simulink model "BMS_OL_Harness_advancedcell"  (R2015b)
settings: Solver=FixedStepDiscrete  StartTime=0.0  StopTime=660  FixedStep=BMSk_stepSize  RelTol=1e-3
undefined symbols (not defined in the file): BMSc_airTemperature, BMSc_cabinTemperature, BMSk_stepSize
settings Model: PauseTimes=22  Creator=ms2zwt  LastModifiedBy=nctzv8
settings ConfigSet: Description=OpenECU configuration set for code generation under RTW-EC.
settings SolverCC: PositivePriorityOrder=on
settings DataIOCC: SaveFormat=Array  SignalLoggingSaveFormat=ModelDataLogs
settings OptimizationCC: DefaultParameterBehavior=Inlined  InlineInvariantSignals=on  ExpressionDepthLimit=2147483647  StateBitsets=on  DataBitsets=on  ZeroExternalMemoryAtStartup=off  ZeroInternalMemoryAtStartup=off  NoFixptDivByZeroProtection=on  EfficientFloat2IntCast=on  OptimizeModelRefInitCode=on  LifeSpan=1
settings DebuggingCC: SaveWithParameterizedLinksMsg=none  UnderspecifiedInitializationDetection=Classic  MergeDetectMultiDrivingBlocksExec=none  SignalResolutionControl=TryResolveAllWithWarning  MultiTaskDSMMsg=warning  MultiTaskCondExecSysMsg=none  SingleTaskRateTransMsg=error  CheckMatrixSingularityMsg=warning  VectorMatrixConversionMsg=warning  FcnCallInpInsideContextMsg=UseLocalSettings  SignalLabelMismatchMsg=warning  StateNameClashWarn=warning
settings HardwareCC: ProdBitPerPointer=32  ProdLargestAtomicInteger=Long  ProdLargestAtomicFloat=Double  ProdEndianess=BigEndian  ProdWordSize=32  ProdHWDeviceType=Freescale->32-bit PowerPC  TargetIntDivRoundTo=Zero  TargetEndianess=BigEndian  TargetHWDeviceType=Freescale->32-bit PowerPC  ProdEqTarget=off
settings RTWCC: SystemTargetFile=openecu_ert.tlc  MakeCommand=make_rtw optimized_floating_point=1  TemplateMakefile=openecu_ert_r2015b_64.tmf  Description=OpenECU Platform Target (ERT, optimised floating-point code)  RetainRTWFile=on  IncludeHyperlinkInReport=on
settings CodeAppCC: ForceParamTrailComments=on  IgnoreCustomStorageClasses=off  SimulinkDataObjDesc=on  CustomSymbolStrType=$N$R$M  InsertBlockDesc=on  InternalIdentifier=Classic
settings STFCustomTargetCC: TargetLibSuffix=.a  GenerateSampleERTMain=on  ConcurrentExecutionCompliant=off  IncludeMdlTerminateFcn=off  GeneratePreprocessorConditionals=Use local settings  CombineOutputUpdateFcns=on  IncludeFileDelimiter=UseQuote  ERTCustomFileBanners=on  SupportContinuousTime=off  MATLABClassNameForMDSCustomization=Simulink.SoftwareTarget.ERTCustomization  CPPClassGenCompliant=off  GRTInterface=off  SystemTargetFile=openecu_ert.tlc
settings ERTTargetCC: GenerateSampleERTMain=on  ParMdlRefBuildCompliant=off  CompOptLevelCompliant=off  ConcurrentExecutionCompliant=off  IncludeMdlTerminateFcn=off  ERTFirstTimeCompliant=off  IncludeFileDelimiter=UseQuote  SupportNonInlinedSFcns=on  ModelStepFunctionPrototypeControlCompliant=off  CPPClassGenCompliant=off  UseToolchainInfoCompliant=off  ExtModeMexFile=noextcomm  InlinedParameterPlacement=NonHierarchical  ERTSrcFileBannerTemplate=oe_code_c_template.cgt  ERTHdrFileBannerTemplate=oe_code_h_template.cgt  ERTDataSrcFileTemplate=oe_data_c_template.cgt  ERTDataHdrFileTemplate=oe_data_h_template.cgt  ERTCustomFileTemplate=example_file_process.tlc  GlobalDataDefinition=InSeparateSourceFile  GlobalDataReference=InSeparateHeaderFile  EnableUserReplacementTypes=on

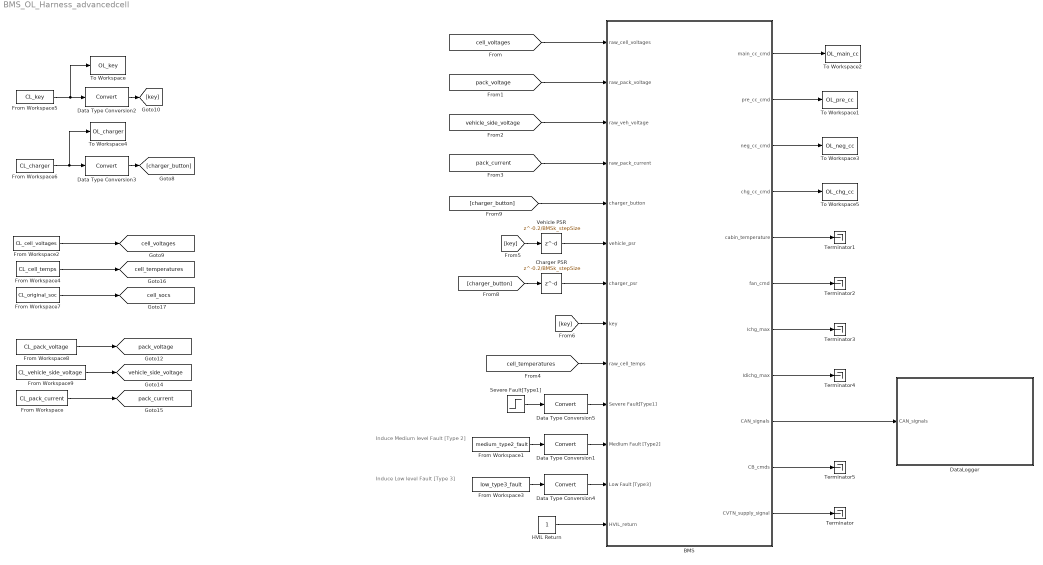
== system BMS_OL_Harness_advancedcell ==
  note: Induce Medium level Fault
      | [Type 2]
  note: Induce Low level Fault
      | [Type 3]
  BMS : Subsystem
  Charger PSR : Delay  DelayLength=0.2/BMSk_stepSize
  Data Type Conversion{1..5} (5 alike) : DataTypeConversion
  DataLogger : Subsystem
  From Workspace : FromWorkspace  VariableName=CL_pack_current  SampleTime=BMSk_stepSize
  From Workspace1 : FromWorkspace  VariableName=medium_type2_fault  SampleTime=BMSk_stepSize
  From Workspace2 : FromWorkspace  VariableName=CL_cell_voltages  SampleTime=BMSk_stepSize
  From Workspace3 : FromWorkspace  VariableName=low_type3_fault  SampleTime=BMSk_stepSize
  From Workspace4 : FromWorkspace  VariableName=CL_cell_temps  SampleTime=BMSk_stepSize
  From Workspace5 : FromWorkspace  VariableName=CL_key  SampleTime=BMSk_stepSize
  From Workspace6 : FromWorkspace  VariableName=CL_charger  SampleTime=BMSk_stepSize
  From Workspace7 : FromWorkspace  VariableName=CL_original_soc  SampleTime=BMSk_stepSize
  From Workspace8 : FromWorkspace  VariableName=CL_pack_voltage  SampleTime=BMSk_stepSize
  From Workspace9 : FromWorkspace  VariableName=CL_vehicle_side_voltage  SampleTime=BMSk_stepSize
  HVIL Return : Constant  OutDataTypeStr=double  SampleTime=-1
  Severe Fault[Type1] : Step  Time=0  After=0
  Terminator{,1..5} (6 alike) : Terminator
  To Workspace : ToWorkspace  VariableName=OL_key  SaveFormat=Timeseries  SampleTime=-1
  To Workspace1 : ToWorkspace  VariableName=OL_pre_cc  SaveFormat=Timeseries  SampleTime=-1
  To Workspace2 : ToWorkspace  VariableName=OL_main_cc  SaveFormat=Timeseries  SampleTime=-1
  To Workspace3 : ToWorkspace  VariableName=OL_neg_cc  SaveFormat=Timeseries  SampleTime=-1
  To Workspace4 : ToWorkspace  VariableName=OL_charger  SaveFormat=Timeseries  SampleTime=-1
  To Workspace5 : ToWorkspace  VariableName=OL_chg_cc  SaveFormat=Timeseries  SampleTime=-1
  Vehicle PSR : Delay  DelayLength=0.2/BMSk_stepSize
  tag scope: cell_socs=global, cell_temperatures=global, cell_voltages=global, pack_current=global, pack_voltage=global, vehicle_side_voltage=global
  wires:
  [cell_temperatures] -> BMS/9(raw_cell_temps)
  Vehicle PSR/1 -> BMS/6(vehicle_psr)
  [key] -> Vehicle PSR/1
  [key] -> BMS/8(key)
  [charger_button] -> BMS/5(charger_button)
  Charger PSR/1 -> BMS/7(charger_psr)
  [charger_button] -> Charger PSR/1
  BMS/4(chg_cc_cmd) -> To Workspace5/1
  BMS/3(neg_cc_cmd) -> To Workspace3/1
  BMS/1(main_cc_cmd) -> To Workspace2/1
  Data Type Conversion2/1 -> [key]
  Data Type Conversion4/1 -> BMS/12(Low Fault [Type3])
  From Workspace1/1 -> Data Type Conversion1/1
  Data Type Conversion5/1 -> BMS/10(Severe Fault[Type1])
  [pack_current] -> BMS/4(raw_pack_current)
  [vehicle_side_voltage] -> BMS/3(raw_veh_voltage)
  [pack_voltage] -> BMS/2(raw_pack_voltage)
  [cell_voltages] -> BMS/1(raw_cell_voltages)
  BMS/9(CAN_signals) -> DataLogger/1(CAN_signals)
  BMS/2(pre_cc_cmd) -> To Workspace1/1
  Data Type Conversion3/1 -> [charger_button]
  From Workspace5/1 -> To Workspace/1, Data Type Conversion2/1
  From Workspace6/1 -> To Workspace4/1, Data Type Conversion3/1
  Data Type Conversion1/1 -> BMS/11(Medium Fault [Type2])
  BMS/11(CVTN_supply_signal) -> Terminator/1
  HVIL Return/1 -> BMS/13(HVIL_return)
  From Workspace3/1 -> Data Type Conversion4/1
  BMS/5(cabin_temperature) -> Terminator1/1
  BMS/6(fan_cmd) -> Terminator2/1
  BMS/7(Ichg_max) -> Terminator3/1
  BMS/8(Idichg_max) -> Terminator4/1
  BMS/10(CB_cmds) -> Terminator5/1
  From Workspace2/1 -> [cell_voltages]
  From Workspace4/1 -> [cell_temperatures]
  From Workspace7/1 -> [cell_socs]
  From Workspace8/1 -> [pack_voltage]
  From Workspace9/1 -> [vehicle_side_voltage]
  From Workspace/1 -> [pack_current]
  Severe Fault[Type1]/1 -> Data Type Conversion5/1

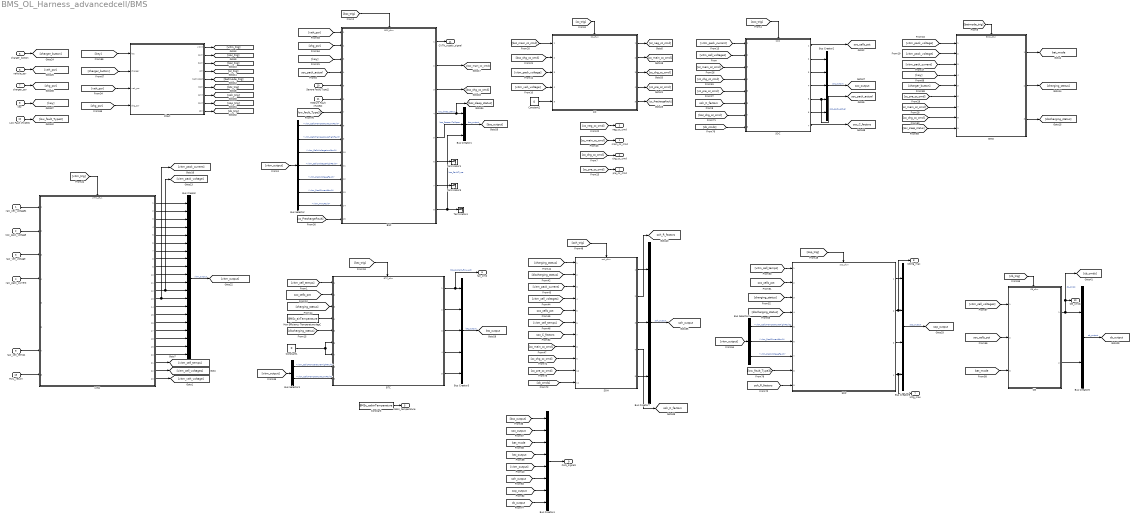
== system BMS_OL_Harness_advancedcell/BMS ==
  raw_cell_voltages : Inport
  raw_pack_voltage : Inport  Port=2
  raw_veh_voltage : Inport  Port=3
  raw_pack_current : Inport  Port=4
  charger_button : Inport  Port=5  OutDataTypeStr=uint8
  vehicle_psr : Inport  Port=6
  charger_psr : Inport  Port=7
  key : Inport  Port=8  OutDataTypeStr=uint8
  raw_cell_temps : Inport  Port=9
  Severe Fault[Type1] : Inport  Port=10
  Medium Fault [Type2] : Inport  Port=11
  Low Fault [Type3] : Inport  Port=12
  HVIL_return : Inport  Port=13  OutDataTypeStr=double
  BMO : ModelReference  ModelNameDialog=BMO_sfun.slx  SimulationMode=Normal  Variant=on  ModelReferenceVersion=1.4  CopyOfModelName=BMO_sfun.slx  TriggerPortName=Trigger  TriggerPortTriggerType=function-call  TriggerPortStatesWhenEnabling=held
  BSC : ModelReference  ModelNameDialog=BSC_sfun.slx  SimulationMode=Normal  Variant=on  ModelReferenceVersion=1.3  CopyOfModelName=BSC_sfun.slx  TriggerPortName=Trigger  TriggerPortTriggerType=function-call  TriggerPortStatesWhenEnabling=held
  BTC : ModelReference  ModelNameDialog=BTC_sfun.slx  SimulationMode=Normal  Variant=on  ModelReferenceVersion=1.3  CopyOfModelName=BTC_sfun.slx  TriggerPortName=Trigger  TriggerPortTriggerType=function-call  TriggerPortStatesWhenEnabling=held
  Bus Creator : BusCreator  Inputs=20
  Bus Creator1 : BusCreator  Inputs=3
  Bus Creator2 : BusCreator  Inputs=5
  Bus Creator3 : BusCreator  Inputs=5
  Bus Creator4 : BusCreator  Inputs=8
  Bus Creator5 : BusCreator  Inputs=4
  Bus Creator6 : BusCreator  Inputs=2
  Bus Creator7 : BusCreator  Inputs=3
  Bus Selector : BusSelector  OutputSignals=vitm_CellsTemperatureLowFault,vitm_CellsTemperatureHighFault,vitm_CellsVoltageLowFault,vitm_CellsVoltageHighFault,vitm_PackVoltageFault,vitm_PackCurrentFault,vitm_HVILFault
  Bus Selector1 : BusSelector  OutputSignals=vitm_CellsTemperatureHighFault,vitm_CellsTemperatureLowFault
  Bus Selector2 : BusSelector  OutputSignals=vitm_CellsTemperatureHighFault,vitm_PackCurrentFault,vitm_PackVoltageFault
  CB : ModelReference  ModelNameDialog=CB_sfun.slx  SimulationMode=Normal  Variant=on  ModelReferenceVersion=1.3  CopyOfModelName=CB_sfun.slx  TriggerPortName=Trigger  TriggerPortTriggerType=function-call  TriggerPortStatesWhenEnabling=held
  CC : ModelReference  ModelNameDialog=CC_sfun.slx  SimulationMode=Normal  Variant=on  ModelReferenceVersion=1.2  CopyOfModelName=CC_sfun.slx  TriggerPortName=Trigger  TriggerPortTriggerType=function-call  TriggerPortStatesWhenEnabling=held
  Chart : Stateflow chart  TreatAsAtomicUnit=on
  Constant : Constant  Value=BMSc_cabinTemperature  SampleTime=BMSk_stepSize
  Constant1 : Constant  Value=0  OutDataTypeStr=boolean  SampleTime=-1
  Constant2 : Constant  Value=0  OutDataTypeStr=double  SampleTime=-1
  Max Efficiency Temperature degC : Constant  Value=BMSc_airTemperature  SampleTime=BMSk_stepSize
  SOC : ModelReference  ModelNameDialog=SOC.slx  SimulationMode=Normal  Variant=on  ModelReferenceVersion=1.297  CopyOfModelName=SOC.slx  TriggerPortName=Trigger  TriggerPortTriggerType=function-call  TriggerPortStatesWhenEnabling=held
  SOH : ModelReference  ModelNameDialog=soh_sfun.slx  SimulationMode=Normal  Variant=on  ModelReferenceVersion=1.3  CopyOfModelName=soh_sfun.slx  TriggerPortName=Trigger  TriggerPortTriggerType=function-call  TriggerPortStatesWhenEnabling=held
  SOP : ModelReference  ModelNameDialog=sop_sfun.slx  SimulationMode=Normal  Variant=on  ModelReferenceVersion=1.4  CopyOfModelName=sop_sfun.slx  TriggerPortName=Trigger  TriggerPortTriggerType=function-call  TriggerPortStatesWhenEnabling=held
  Terminator1 : Terminator
  Terminator3 : Terminator
  Terminator4 : Terminator
  VITM : ModelReference  ModelNameDialog=VITM_sfun.slx  SimulationMode=Normal  Variant=on  ModelReferenceVersion=1.3  CopyOfModelName=VITM_sfun.slx  TriggerPortName=Trigger  TriggerPortTriggerType=function-call  TriggerPortStatesWhenEnabling=held
  main_cc_cmd : Outport
  pre_cc_cmd : Outport  Port=2
  neg_cc_cmd : Outport  Port=3
  chg_cc_cmd : Outport  Port=4
  cabin_temperature : Outport  Port=5
  fan_cmd : Outport  Port=6
  Ichg_max : Outport  Port=7
  Idichg_max : Outport  Port=8
  CAN_signals : Outport  Port=9
  CB_cmds : Outport  Port=10
  CVTN_supply_signal : Outport  Port=11
  tag scope: bat_mode=global, btc_output=global, cb_output=global, soc_C_factors=global, soc_cells_pct=global, soc_output=global, soc_pack_actual=global, soh_C_factors=global, soh_R_factors=global, soh_output=global, sop_output=global
  wires:
  SOC/1 -> [soc_cells_pct]
  [vitm_pack_voltage] -> BMO/1
  BMO/1 -> [bat_mode]
  [vitm_cell_voltages] -> SOC/2
  Chart/1(vitm()) -> [vitm_trig]
  Chart/2(soc()) -> [soc_trig]
  Chart/3(bsc()) -> [bsc_trig]
  Chart/4(cc()) -> [cc_trig]
  Chart/5(batmode()) -> [batmode_trig]
  [soc_trig] -> SOC/Trigger
  [batmode_trig] -> BMO/Trigger
  [cc_trig] -> CC/Trigger
  Constant/1 -> cabin_temperature/1
  Max Efficiency Temperature degC/1 -> BTC/4
  [vitm_cell_temps] -> BTC/1
  [soc_cells_pct] -> BTC/2
  BMO/2 -> [charging_status]
  BMO/3 -> [discharging_status]
  [charging_status] -> BTC/3
  [discharging_status] -> BTC/5
  Constant1/1 -> BTC/6, BTC/7
  raw_cell_voltages/1 -> VITM/1
  [vitm_pack_current] -> SOC/1
  [vitm_pack_current] -> BMO/3
  [vitm_pack_voltage] -> BMO/2
  [bsc_main_cc_cmd] -> CC/1
  [bsc_chg_cc_cmd] -> CC/2
  CC/1 -> [cc_neg_cc_cmd]
  CC/2 -> [cc_main_cc_cmd]
  CC/3 -> [cc_chg_cc_cmd]
  CC/4 -> [cc_pre_cc_cmd]
  [cc_neg_cc_cmd] -> neg_cc_cmd/1
  [cc_main_cc_cmd] -> main_cc_cmd/1
  [cc_chg_cc_cmd] -> chg_cc_cmd/1
  [cc_pre_cc_cmd] -> pre_cc_cmd/1
  [cc_main_cc_cmd] -> SOC/3
  Chart/6(btc()) -> [btc_trig]
  VITM/1 -> Bus Creator/1
  VITM/2 -> Bus Creator/2
  VITM/3 -> Bus Creator/3
  VITM/4 -> Bus Creator/4
  VITM/5 -> Bus Creator/5
  VITM/6 -> Bus Creator/6
  VITM/7 -> Bus Creator/7
  VITM/8 -> Bus Creator/8
  VITM/9 -> Bus Creator/9
  VITM/10 -> Bus Creator/10
  VITM/11 -> Bus Creator/11
  VITM/12 -> [vitm_pack_voltage], Bus Creator/12
  VITM/13 -> [vitm_pack_current], Bus Creator/13
  VITM/14 -> Bus Creator/14
  VITM/15 -> Bus Creator/15
  VITM/16 -> Bus Creator/16
  VITM/17 -> Bus Creator/17
  VITM/18 -> Bus Creator/18
  VITM/19 -> Bus Creator/19
  Bus Creator/1 -> [vitm_output]  "vitm_output"
  [vitm_output] -> Bus Selector/1
  [btc_trig] -> BTC/Trigger
  raw_pack_voltage/1 -> VITM/2
  raw_pack_current/1 -> VITM/4
  raw_cell_temps/1 -> VITM/7
  CC/5 -> [cc_PrechargeFault]
  raw_veh_voltage/1 -> VITM/3
  charger_button/1 -> [charger_button]
  vehicle_psr/1 -> [veh_psr]
  [veh_psr] -> Chart/3(veh_psr)
  [vitm_output] -> Bus Selector1/1
  Bus Selector1/1 -> BTC/8  "<vitm_CellsTemperatureHighFault>"
  Bus Selector1/2 -> BTC/9  "<vitm_CellsTemperatureLowFault>"
  Bus Creator1/1 -> [bsc_output]  "bsc_output"
  SOC/2 -> Bus Creator2/1
  SOC/3 -> Bus Creator2/2
  SOC/4 -> Bus Creator2/3
  SOC/5 -> Bus Creator2/4, [soc_pack_actual]  "soc_pack_actual"
  SOC/6 -> Bus Creator2/5
  Bus Creator2/1 -> [soc_output]  "soc_output"
  BTC/1 -> fan_cmd/1, Bus Creator3/1  "btc_coolant_flow_pct"
  BTC/2 -> Bus Creator3/2
  BTC/3 -> Bus Creator3/3
  BTC/4 -> Bus Creator3/4
  BTC/5 -> Bus Creator3/5
  Bus Creator3/1 -> [btc_output]  "btc_output"
  [bsc_output] -> Bus Creator4/1
  [soc_output] -> Bus Creator4/2
  [bat_mode] -> Bus Creator4/3
  [btc_output] -> Bus Creator4/4
  [vitm_output] -> Bus Creator4/5
  Bus Creator4/1 -> CAN_signals/1
  [charging_status] -> SOH/1
  [discharging_status] -> SOH/2
  [vitm_pack_current] -> SOH/3
  [vitm_cell_voltages] -> SOH/4
  [soc_cells_pct] -> SOH/5
  [vitm_cell_temps] -> SOH/6
  Chart/7(soh()) -> [soh_trig]
  Chart/8(sop()) -> [sop_trig]
  [vitm_cell_temps] -> SOP/1
  [soc_cells_pct] -> SOP/2
  [charging_status] -> SOP/3
  [discharging_status] -> SOP/4
  [vitm_output] -> Bus Selector2/1
  Bus Selector2/1 -> SOP/5  "<vitm_CellsTemperatureHighFault>"
  Bus Selector2/2 -> SOP/6  "<vitm_PackCurrentFault>"
  Bus Selector2/3 -> SOP/7  "<vitm_PackVoltageFault>"
  Chart/9(cb()) -> [cb_trig]
  [cb_trig] -> CB/Trigger
  [soc_cells_pct] -> CB/2
  [vitm_cell_voltages] -> CB/1
  [bat_mode] -> CB/3
  SOP/1 -> Bus Creator5/1
  SOP/2 -> Bus Creator5/2, Idichg_max/1
  SOP/3 -> Bus Creator5/3
  SOP/4 -> Ichg_max/1, Bus Creator5/4
  Bus Creator5/1 -> [sop_output]  "sop_output"
  [cc_pre_cc_cmd] -> SOC/5
  [cc_chg_cc_cmd] -> SOC/4
  [sop_output] -> Bus Creator4/7
  CB/2 -> Bus Creator6/2
  charger_psr/1 -> [chg_psr]
  [chg_psr] -> Chart/4(chg_psr)
  key/1 -> [key]
  [charger_button] -> Chart/2(charger)
  [key] -> Chart/1(key)
  [cc_pre_cc_cmd] -> BMO/6
  [cc_main_cc_cmd] -> BMO/7
  [cc_chg_cc_cmd] -> BMO/8
  [bsc_sleep_status] -> BMO/9
  [key] -> BMO/4
  [charger_button] -> BMO/5
  [vitm_pack_voltage] -> CC/3
  [vitm_veh_voltage] -> CC/4
  Constant2/1 -> CC/5
  SOC/7 -> [soc_C_factors]
  [soc_C_factors] -> SOH/7
  [soh_C_factors] -> SOC/6
  [bsc_chg_cc_cmd] -> SOC/7
  CB/1 -> Bus Creator6/1, [cb_cmds], CB_cmds/1  "cb_cmds"
  [cc_main_cc_cmd] -> SOH/8
  [cc_pre_cc_cmd] -> SOH/10
  [cc_chg_cc_cmd] -> SOH/9
  [cb_cmds] -> SOC/8
  [cb_cmds] -> SOH/11
  Bus Creator6/1 -> [cb_output]  "cb_output"
  [cb_output] -> Bus Creator4/8
  SOH/1 -> Bus Creator7/1
  SOH/3 -> Bus Creator7/2
  SOH/5 -> Bus Creator7/3
  SOH/2 -> [soh_R_factors]
  SOH/4 -> [soh_C_factors]
  Bus Creator7/1 -> [soh_output]  "soh_output"
  [soh_output] -> Bus Creator4/6
  HVIL_return/1 -> VITM/8
  VITM/20 -> Bus Creator/20
  VITM/21 -> [vitm_cell_temps]
  VITM/22 -> [vitm_cell_voltages]
  VITM/23 -> [vitm_veh_voltage]
  [soh_R_factors] -> SOP/9
  Low Fault [Type3]/1 -> [low_fault_Type3]
  [low_fault_Type3] -> SOP/8
  BSC/4 -> [bsc_sleep_status], Bus Creator1/1  "bsc_sleep_status"
  [veh_psr] -> BSC/1
  [chg_psr] -> BSC/2
  [key] -> BSC/3
  [soc_pack_actual] -> BSC/4
  Severe Fault[Type1]/1 -> BSC/5
  Medium Fault [Type2]/1 -> BSC/6
  [low_fault_Type3] -> BSC/7
  Bus Selector/1 -> BSC/8  "<vitm_CellsTemperatureLowFault>"
  Bus Selector/2 -> BSC/9  "<vitm_CellsTemperatureHighFault>"
  Bus Selector/3 -> BSC/10  "<vitm_CellsVoltageLowFault>"
  Bus Selector/4 -> BSC/11  "<vitm_CellsVoltageHighFault>"
  Bus Selector/5 -> BSC/12  "<vitm_PackVoltageFault>"
  Bus Selector/6 -> BSC/13  "<vitm_PackCurrentFault>"
  Bus Selector/7 -> BSC/14  "<vitm_HVILFault>"
  [cc_PrechargeFault] -> BSC/15
  BSC/1 -> CVTN_supply_signal/1
  BSC/2 -> [bsc_main_cc_cmd]
  BSC/3 -> [bsc_chg_cc_cmd]
  BSC/5 -> Bus Creator1/2  "bsc_ReasonToOpen"
  BSC/7 -> Terminator3/1
  BSC/8 -> Bus Creator1/3, Terminator4/1  "bsc_FaultType"
  [bsc_trig] -> BSC/Trigger
  BSC/6 -> Terminator1/1
  [soh_trig] -> SOH/Trigger
  [sop_trig] -> SOP/Trigger
  [vitm_trig] -> VITM/Trigger

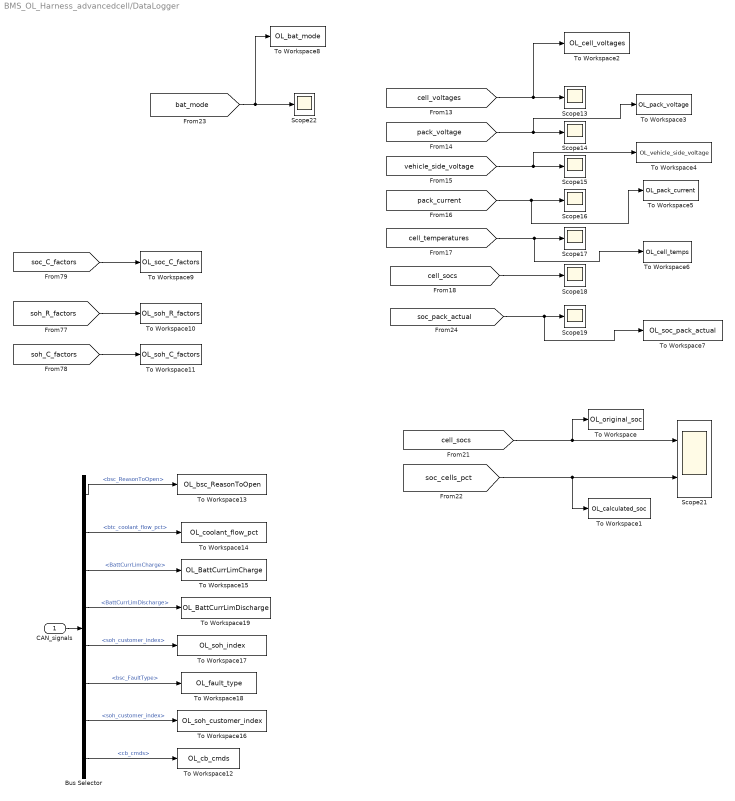
== system BMS_OL_Harness_advancedcell/DataLogger ==
  CAN_signals : Inport
  Bus Selector : BusSelector  OutputSignals=bsc_output.bsc_ReasonToOpen,btc_output.btc_coolant_flow_pct,sop_output.BattCurrLimCharge,sop_output.BattCurrLimDischarge,soh_output.soh_customer_index,bsc_output.bsc_FaultType,soh_output.soh_customer_index,cb_output.cb_cmds
  Scope{13..19,22} (8 alike) : Scope
  Scope21 : Scope  NumInputPorts=2
  To Workspace : ToWorkspace  VariableName=OL_original_soc  SaveFormat=Timeseries  SampleTime=-1
  To Workspace1 : ToWorkspace  VariableName=OL_calculated_soc  SaveFormat=Timeseries  SampleTime=-1
  To Workspace10 : ToWorkspace  VariableName=OL_soh_R_factors  SaveFormat=Timeseries  SampleTime=-1
  To Workspace11 : ToWorkspace  VariableName=OL_soh_C_factors  SaveFormat=Timeseries  SampleTime=-1
  To Workspace12 : ToWorkspace  VariableName=OL_cb_cmds  SaveFormat=Timeseries  SampleTime=-1
  To Workspace13 : ToWorkspace  VariableName=OL_bsc_ReasonToOpen  SaveFormat=Timeseries  SampleTime=-1
  To Workspace14 : ToWorkspace  VariableName=OL_coolant_flow_pct  SaveFormat=Timeseries  SampleTime=-1
  To Workspace15 : ToWorkspace  VariableName=OL_BattCurrLimCharge  SaveFormat=Timeseries  SampleTime=-1
  To Workspace16 : ToWorkspace  VariableName=OL_soh_customer_index  SaveFormat=Timeseries  SampleTime=-1
  To Workspace17 : ToWorkspace  VariableName=OL_soh_index  SaveFormat=Timeseries  SampleTime=-1
  To Workspace18 : ToWorkspace  VariableName=OL_fault_type  SaveFormat=Timeseries  SampleTime=-1
  To Workspace19 : ToWorkspace  VariableName=OL_BattCurrLimDischarge  SaveFormat=Timeseries  SampleTime=-1
  To Workspace2 : ToWorkspace  VariableName=OL_cell_voltages  SaveFormat=Timeseries  SampleTime=-1
  To Workspace3 : ToWorkspace  VariableName=OL_pack_voltage  SaveFormat=Timeseries  SampleTime=-1
  To Workspace4 : ToWorkspace  VariableName=OL_vehicle_side_voltage  SaveFormat=Timeseries  SampleTime=-1
  To Workspace5 : ToWorkspace  VariableName=OL_pack_current  SaveFormat=Timeseries  SampleTime=-1
  To Workspace6 : ToWorkspace  VariableName=OL_cell_temps  SaveFormat=Timeseries  SampleTime=-1
  To Workspace7 : ToWorkspace  VariableName=OL_soc_pack_actual  SaveFormat=Timeseries  SampleTime=-1
  To Workspace8 : ToWorkspace  VariableName=OL_bat_mode  SaveFormat=Timeseries  SampleTime=-1
  To Workspace9 : ToWorkspace  VariableName=OL_soc_C_factors  SaveFormat=Timeseries  SampleTime=-1
  wires:
  [cell_voltages] -> To Workspace2/1, Scope13/1
  [pack_voltage] -> To Workspace3/1, Scope14/1
  [vehicle_side_voltage] -> To Workspace4/1, Scope15/1
  [pack_current] -> To Workspace5/1, Scope16/1
  [cell_temperatures] -> To Workspace6/1, Scope17/1
  [cell_socs] -> Scope18/1
  [cell_socs] -> To Workspace/1, Scope21/1
  [bat_mode] -> To Workspace8/1, Scope22/1
  [soc_cells_pct] -> To Workspace1/1, Scope21/2
  [soc_pack_actual] -> To Workspace7/1, Scope19/1
  [soc_C_factors] -> To Workspace9/1
  [soh_C_factors] -> To Workspace11/1
  [soh_R_factors] -> To Workspace10/1
  CAN_signals/1 -> Bus Selector/1
  Bus Selector/1 -> To Workspace13/1  "<bsc_ReasonToOpen>"
  Bus Selector/2 -> To Workspace14/1  "<btc_coolant_flow_pct>"
  Bus Selector/3 -> To Workspace15/1  "<BattCurrLimCharge>"
  Bus Selector/7 -> To Workspace16/1  "<soh_customer_index>"
  Bus Selector/6 -> To Workspace18/1  "<bsc_FaultType>"
  Bus Selector/5 -> To Workspace17/1  "<soh_customer_index>"
  Bus Selector/4 -> To Workspace19/1  "<BattCurrLimDischarge>"
  Bus Selector/8 -> To Workspace12/1  "<cb_cmds>"

== stateflow chart BMS_OL_Harness_advancedcell/BMS/Chart ==
  state main_chg
    (default) -> (junction 607)
    main_chg -> (junction 607) [order 1]
    (junction 607) -> (junction 606) : {vitm;}
    (junction 606) -> (junction 597) : {soc;}
    (junction 597) -> (junction 612) : {bsc;}
    (junction 612) -> (junction 598) : {soh;}
    (junction 598) -> (junction 604) : {cc;}
    (junction 604) -> (junction 605) : {batmode;}
    (junction 605) -> (junction 592) : {btc;}
    (junction 592) -> (junction 593) : {sop;}
    (junction 593) -> (junction 594) : {cb;}
  state main_key
    (default) -> (junction 544)
    main_key -> (junction 544) [order 1]
    (junction 544) -> (junction 543) : {vitm;}
    (junction 543) -> (junction 534) : {soc;}
    (junction 534) -> (junction 549) : {bsc;}
    (junction 549) -> (junction 535) : {soh;}
    (junction 535) -> (junction 541) : {cc;}
    (junction 541) -> (junction 542) : {batmode;}
    (junction 542) -> (junction 529) : {btc;}
    (junction 529) -> (junction 530) : {sop;}
    (junction 530) -> (junction 531) : {cb;}
  state init_key
    (default) -> (junction 81)
    init_key -> (junction 81) [order 1]
    (junction 81) -> (junction 83) : {vitm;}
    (junction 83) -> (junction 89) : {soc;}
    (junction 89) -> (junction 527) : {bsc;}
    (junction 527) -> (junction 82) : {soh;}
    (junction 82) -> (junction 85) : {cc;}
    (junction 85) -> (junction 87) : {batmode;}
    (junction 87) -> (junction 158) : {btc;}
    (junction 158) -> (junction 195) : {sop;}
    (junction 195) -> (junction 236) : {cb;}
  state init_chg
    (default) -> (junction 586)
    init_chg -> (junction 586) [order 1]
    (junction 586) -> (junction 585) : {vitm;}
    (junction 585) -> (junction 576) : {soc;}
    (junction 576) -> (junction 591) : {bsc;}
    (junction 591) -> (junction 577) : {soh;}
    (junction 577) -> (junction 583) : {cc;}
    (junction 583) -> (junction 584) : {batmode;}
    (junction 584) -> (junction 571) : {btc;}
    (junction 571) -> (junction 572) : {sop;}
    (junction 572) -> (junction 573) : {cb;}
  state no_power
    entry:
    end_count =0;
  state end_key
    exit:
    end_count = end_count +1;
    (default) -> (junction 565)
    end_key -> (junction 565) [order 1]
    (junction 565) -> (junction 564) : {vitm;}
    (junction 564) -> (junction 555) : {soc;}
    (junction 555) -> (junction 570) : {bsc;}
    (junction 570) -> (junction 556) : {soh;}
    (junction 556) -> (junction 562) : {cc;}
    (junction 562) -> (junction 563) : {batmode;}
    (junction 563) -> (junction 550) : {btc;}
    (junction 550) -> (junction 551) : {sop;}
    (junction 551) -> (junction 552) : {cb;}
  state end_chg
    exit:
    end_count = end_count +1;
    (default) -> (junction 628)
    end_chg -> (junction 628) [order 1]
    (junction 628) -> (junction 627) : {vitm;}
    (junction 627) -> (junction 618) : {soc;}
    (junction 618) -> (junction 633) : {bsc;}
    (junction 633) -> (junction 619) : {soh;}
    (junction 619) -> (junction 625) : {cc;}
    (junction 625) -> (junction 626) : {batmode;}
    (junction 626) -> (junction 613) : {btc;}
    (junction 613) -> (junction 614) : {sop;}
    (junction 614) -> (junction 615) : {cb;}
  (default) -> no_power
  no_power -> init_chg [order 2] : [charger > 0.5]
  no_power -> init_key [order 1] : [key > 0.5]
  end_chg -> no_power [order 2]
  end_key -> no_power [order 2]
  init_key -> main_key [order 1]
  init_chg -> main_chg [order 1]
  main_chg -> end_chg [order 1] : [chg_psr < 0.5]
  main_key -> end_key [order 1] : [veh_psr < 0.5]
  end_key -> end_key [order 1] : [end_count < 10]
  end_chg -> end_chg [order 1] : [end_count < 10]
  data: key input; charger input; veh_psr input; end_count local double =0; chg_psr input
  events: vitm output FUNCTION_CALL_EVENT; soc output FUNCTION_CALL_EVENT; bsc output FUNCTION_CALL_EVENT; cc output FUNCTION_CALL_EVENT; batmode output FUNCTION_CALL_EVENT; btc output FUNCTION_CALL_EVENT; soh output FUNCTION_CALL_EVENT; sop output FUNCTION_CALL_EVENT; cb output FUNCTION_CALL_EVENT
